simulink subsystem "Find_Curvature"  (R2023b)
settings: Solver=VariableStepAuto  StartTime=0.0  StopTime=10.0  RelTol=1e-3
settings Model: Creator=FIRSTMentor  LastModifiedBy=FIRSTMentor

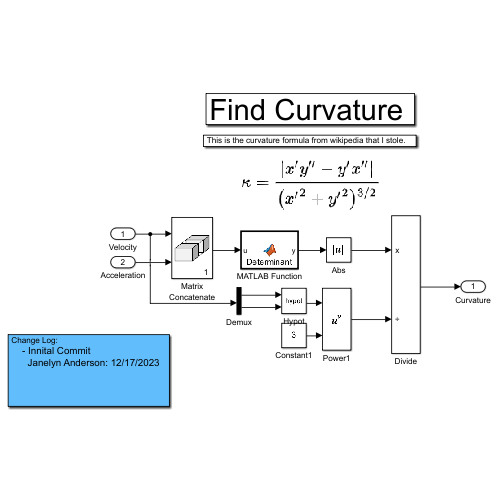
[thumbnail: Simulink's stored preview of the top-level diagram]
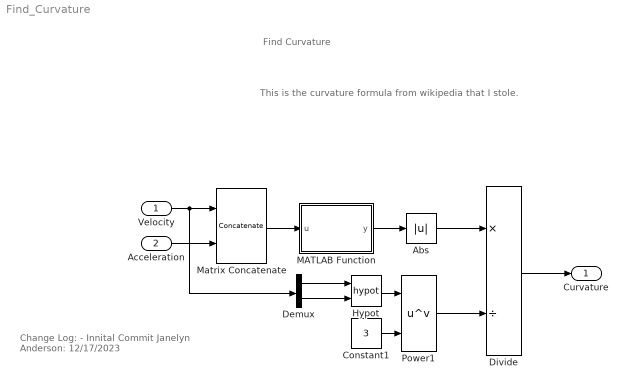
== system Find_Curvature ==
  note: Change Log:
      | - Innital Commit
      | Janelyn Anderson: 12/17/2023
  note: Find Curvature
  note: This is the curvature formula from wikipedia that I stole.
  Velocity : Inport  PortDimensions=[1 2]
  Acceleration : Inport  Port=2  PortDimensions=[1 2]
  Abs : Abs  SaturateOnIntegerOverflow=off
  Constant1 : Constant  Value=3
  Demux : Demux  Outputs=2
  Divide : Product  Inputs=*/
  Hypot : Math  Operator=hypot
  MATLAB Function : MATLAB Function  TreatAsAtomicUnit=on
  Matrix Concatenate : Concatenate  Mode=Multidimensional array
  Power1 : Math  Operator=pow
  Curvature : Outport  PortDimensions=1
  wires:
  Demux/2 -> Hypot/2
  Power1/1 -> Divide/2
  Demux/1 -> Hypot/1
  Abs/1 -> Divide/1
  Hypot/1 -> Power1/1
  MATLAB Function/1(y) -> Abs/1
  Constant1/1 -> Power1/2
  Matrix Concatenate/1 -> MATLAB Function/1(u)
  Divide/1 -> Curvature/1
  Velocity/1 -> Demux/1, Matrix Concatenate/1
  Acceleration/1 -> Matrix Concatenate/2

== matlab function Find_Curvature/MATLAB Function ==
  data: u input size=[2 2]; y output size=1
function y = Determinant(u)

y = u(1,1)*u(2,2)-u(2,1)*u(1,2);
